simulink model "quarterVehicleMdl"  (R2013a)
settings: Solver=ode45  StartTime=0.0  StopTime=10.0  RelTol=1e-3
values from neighbouring files (symbols this model uses):
  g = 9.81    [abssim1.mat]    (also in abssim2.mat; abssim3.mat; initAbsSim.m)
  m = 9    [abssim1.mat]    (also in abssim2.mat; abssim3.mat; initAbsSim.m)
  Rd = 0.0625    [abssim1.mat]    (also in abssim2.mat; abssim3.mat; initAbsSim.m)
  v0 = 20    [abssim1.mat]    (also in abssim2.mat; abssim3.mat; initAbsSim.m = 5)
libraries: simulink x1
settings Model: Creator=kortetl1  LastModifiedBy=kortetl1

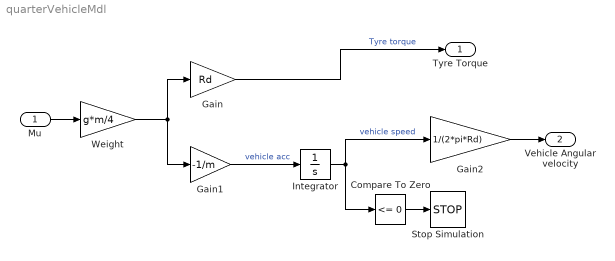
== system quarterVehicleMdl ==
  Mu : Inport
  Compare To Zero : simulink/Logic and Bit Operations/Compare To Zero  relop=<=  OutDataTypeStr=boolean
  Gain : Gain  Gain=Rd
  Gain1 : Gain  Gain=-1/m
  Gain2 : Gain  Gain=1/(2*pi*Rd)
  Integrator : Integrator  InitialCondition=v0
  Stop Simulation : Stop
  Weight : Gain  Gain=g*m/4
  Tyre Torque : Outport
  Vehicle Angular velocity : Outport  Port=2
  wires:
  Weight/1 -> Gain1/1, Gain/1
  Gain/1 -> Tyre Torque/1  "Tyre torque"
  Gain1/1 -> Integrator/1  "vehicle acc"
  Integrator/1 -> Compare To Zero/1, Gain2/1  "vehicle speed"
  Compare To Zero/1 -> Stop Simulation/1
  Mu/1 -> Weight/1
  Gain2/1 -> Vehicle Angular velocity/1
